simulink library "LIB_TF_G_112"  (Simulink 8.6)
settings: Solver=ode45  StartTime=0.0  StopTime=10.0  RelTol=1e-3
PreLoadFcn:
  | if exist('tl_preloadfcn','file'), tl_preloadfcn(gcs,402); end
PostLoadFcn:
  | if exist('tl_postloadfcn','file'), tl_postloadfcn(gcs,402); end
undefined symbols (not defined in the file or in its folder): ddv
libraries: tllib x2
(part 2 of 2)

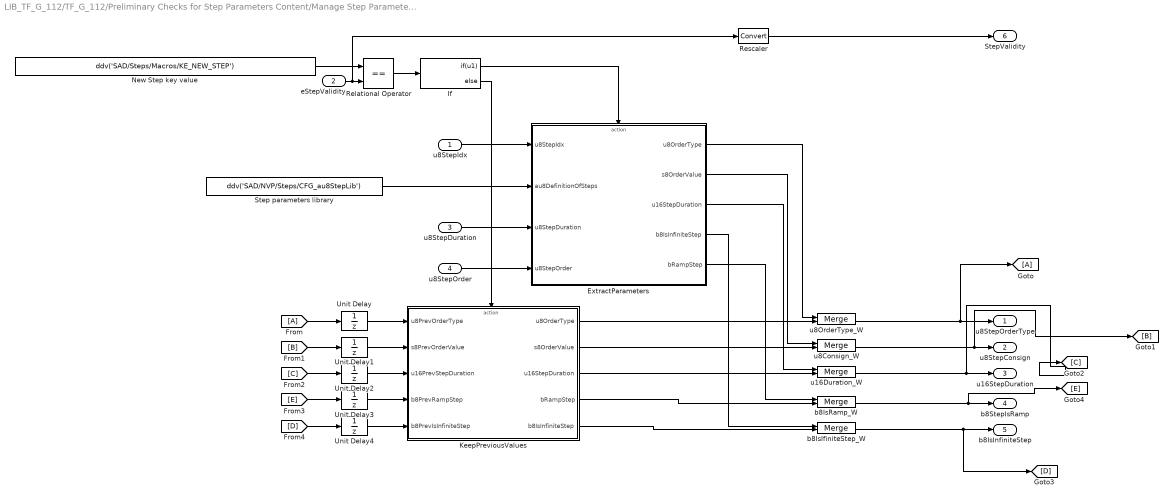
== system LIB_TF_G_112/TF_G_112/Preliminary Checks for Step Parameters Content/Manage Step Parameters ==
  u8StepIdx : Inport
  eStepValidity : Inport  Port=2  PortDimensions=1
  u8StepDuration : Inport  Port=3
  u8StepOrder : Inport  Port=4
  ExtractParameters : Subsystem  RequirementInfo={} %GIDa_f8518a03_50c3_4128_a0d7_e66c9cadc317  TreatAsAtomicUnit=on
  If : If  IfExpression=u1
  KeepPreviousValues : Subsystem  RequirementInfo={} %GIDa_d99f78ca_cceb_45f0_b7aa_f1ab4b729ade  TreatAsAtomicUnit=on
  New Step key value : Constant  Value=ddv('SAD/Steps/Macros/KE_NEW_STEP')  mask(TL_Constant){data={'output',{'variable','SAD/Steps/Macros/KE_NEW_STEP'},'date',738321.40615506948}}
      settings: CopyFcn=if exist('tl_reset_reviewflag','file')==2,tl_reset_reviewflag(gcbh);end  DeleteFcn=if exist('delete_tlblock','file')==2,delete_tlblock(gcbh);end  NameChangeFcn=if exist('rename_tlblock','file')==2,rename_tlblock(gcbh);end  OpenFcn=if exist('tl_open_blockdlg','file')==2,tl_open_blockdlg(gcbh);else,open_system(gcbh,'parameter');end
      mask Help: eval(['if exist(''tl_online_help'',''file'') == 2, tl_online_help(''Topic'',''TL_Constant''),else, web([''jar:file:///'',matlabroot,''/help/toolbox/simulink/help.jar!/slref/' lower(get_param(gcbh,'Blocktype')) '.html''], ''-helpbrowser''),end'])
      mask Display: plot([-0.05, 1.05, NaN, -0.05, 1.05],[.01, .01, NaN, .99, .99])
  Relational Operator : RelationalOperator  Operator===  OutDataTypeStr=boolean  mask(TL_RelationalOperator){data={'date',735951.66826406249}}
      settings: DeleteFcn=if exist('delete_tlblock','file')==2,delete_tlblock(gcbh);end  NameChangeFcn=if exist('rename_tlblock','file')==2,rename_tlblock(gcbh);end  OpenFcn=if exist('tl_open_blockdlg','file')==2,tl_open_blockdlg(gcbh);else,open_system(gcbh,'parameter');end
      mask Help: eval(['if exist(''tl_online_help'',''file'') == 2, tl_online_help(''Topic'',''TL_RelationalOperator''),else, web([''jar:file:///'',matlabroot,''/help/toolbox/simulink/help.jar!/slref/' lower(get_param(gcbh,'Blocktype')) '.html''], ''-helpbrowser''),end'])
      mask Display: plot([-0.05, 1.05, NaN, -0.05, 1.05],[.01, .01, NaN, .99, .99])
  Rescaler : DataTypeConversion  mask(TL_Rescaler){data={'output',{'type','UInt8'},'date',738378.35896812496}}
      settings: DeleteFcn=if exist('delete_tlblock','file')==2,delete_tlblock(gcbh);end  NameChangeFcn=if exist('rename_tlblock','file')==2,rename_tlblock(gcbh);end  OpenFcn=if exist('tl_open_blockdlg','file')==2,tl_open_blockdlg(gcbh);else,open_system(gcbh,'parameter');end
      mask Help: eval(['if exist(''tl_online_help'',''file'') == 2, tl_online_help(''Topic'',''TL_Rescaler''),else, web([''jar:file:///'',matlabroot,''/help/toolbox/simulink/help.jar!/slref/' lower(get_param(gcbh,'Blocktype')) '.html''], ''-helpbrowser''),end'])
      mask Display: plot([-0.1, 1.05, NaN, -0.1, 1.05],[.01, .01, NaN, .99, .99]);
  Step parameters library : Constant  RequirementInfo={} %GIDa_701f29de_2d44_4d45_a297_c60af8fddfb1  Value=ddv('SAD/NVP/Steps/CFG_au8StepLib')  OutDataTypeStr=uint8  SampleTime=-1  mask(TL_Constant){data={'output',{'variable','SAD/NVP/Steps/CFG_au8StepLib'},'date',738321.40645788191}}
      settings: CopyFcn=if exist('tl_reset_reviewflag','file')==2,tl_reset_reviewflag(gcbh);end  DeleteFcn=if exist('delete_tlblock','file')==2,delete_tlblock(gcbh);end  NameChangeFcn=if exist('rename_tlblock','file')==2,rename_tlblock(gcbh);end  OpenFcn=if exist('tl_open_blockdlg','file')==2,tl_open_blockdlg(gcbh);else,open_system(gcbh,'parameter');end
      mask Help: eval(['if exist(''tl_online_help'',''file'') == 2, tl_online_help(''Topic'',''TL_Constant''),else, web([''jar:file:///'',matlabroot,''/help/toolbox/simulink/help.jar!/slref/' lower(get_param(gcbh,'Blocktype')) '.html''], ''-helpbrowser''),end'])
      mask Display: plot([-0.05, 1.05, NaN, -0.05, 1.05],[.01, .01, NaN, .99, .99])
  Unit Delay : UnitDelay  SampleTime=-1  mask(TL_UnitDelay){data={'date',738654.44428931712}}
      settings: CopyFcn=if exist('tl_reset_reviewflag') == 2, tl_reset_reviewflag(gcbh); end  DeleteFcn=if exist('delete_tlblock','file')==2,delete_tlblock(gcbh);end  NameChangeFcn=if exist('rename_tlblock','file')==2,rename_tlblock(gcbh);end  OpenFcn=if exist('tl_open_blockdlg','file')==2,tl_open_blockdlg(gcbh);else,open_system(gcbh,'parameter');end
      mask Help: eval(['if exist(''tl_online_help'',''file'') == 2, tl_online_help(''Topic'',''TL_UnitDelay''),else, web([''jar:file:///'',matlabroot,''/help/toolbox/simulink/help.jar!/slref/' lower(get_param(gcbh,'Blocktype')) '.html''], ''-helpbrowser''),end'])
      mask Display: plot([-0.1, 1.05, NaN, -0.1, 1.05],[.01, .01, NaN, .99, .99]);
  Unit Delay1 : UnitDelay  SampleTime=-1  mask(TL_UnitDelay){data={'date',738654.44460206013}}
      settings: CopyFcn=if exist('tl_reset_reviewflag') == 2, tl_reset_reviewflag(gcbh); end  DeleteFcn=if exist('delete_tlblock','file')==2,delete_tlblock(gcbh);end  NameChangeFcn=if exist('rename_tlblock','file')==2,rename_tlblock(gcbh);end  OpenFcn=if exist('tl_open_blockdlg','file')==2,tl_open_blockdlg(gcbh);else,open_system(gcbh,'parameter');end
      mask Help: eval(['if exist(''tl_online_help'',''file'') == 2, tl_online_help(''Topic'',''TL_UnitDelay''),else, web([''jar:file:///'',matlabroot,''/help/toolbox/simulink/help.jar!/slref/' lower(get_param(gcbh,'Blocktype')) '.html''], ''-helpbrowser''),end'])
      mask Display: plot([-0.1, 1.05, NaN, -0.1, 1.05],[.01, .01, NaN, .99, .99]);
  Unit Delay2 : UnitDelay  SampleTime=-1  mask(TL_UnitDelay){data={'date',738654.44480167818}}
      settings: CopyFcn=if exist('tl_reset_reviewflag') == 2, tl_reset_reviewflag(gcbh); end  DeleteFcn=if exist('delete_tlblock','file')==2,delete_tlblock(gcbh);end  NameChangeFcn=if exist('rename_tlblock','file')==2,rename_tlblock(gcbh);end  OpenFcn=if exist('tl_open_blockdlg','file')==2,tl_open_blockdlg(gcbh);else,open_system(gcbh,'parameter');end
      mask Help: eval(['if exist(''tl_online_help'',''file'') == 2, tl_online_help(''Topic'',''TL_UnitDelay''),else, web([''jar:file:///'',matlabroot,''/help/toolbox/simulink/help.jar!/slref/' lower(get_param(gcbh,'Blocktype')) '.html''], ''-helpbrowser''),end'])
      mask Display: plot([-0.1, 1.05, NaN, -0.1, 1.05],[.01, .01, NaN, .99, .99]);
  Unit Delay3 : UnitDelay  SampleTime=-1  mask(TL_UnitDelay){data={'date',738654.44489355327}}
      settings: CopyFcn=if exist('tl_reset_reviewflag') == 2, tl_reset_reviewflag(gcbh); end  DeleteFcn=if exist('delete_tlblock','file')==2,delete_tlblock(gcbh);end  NameChangeFcn=if exist('rename_tlblock','file')==2,rename_tlblock(gcbh);end  OpenFcn=if exist('tl_open_blockdlg','file')==2,tl_open_blockdlg(gcbh);else,open_system(gcbh,'parameter');end
      mask Help: eval(['if exist(''tl_online_help'',''file'') == 2, tl_online_help(''Topic'',''TL_UnitDelay''),else, web([''jar:file:///'',matlabroot,''/help/toolbox/simulink/help.jar!/slref/' lower(get_param(gcbh,'Blocktype')) '.html''], ''-helpbrowser''),end'])
      mask Display: plot([-0.1, 1.05, NaN, -0.1, 1.05],[.01, .01, NaN, .99, .99]);
  Unit Delay4 : UnitDelay  SampleTime=-1  mask(TL_UnitDelay){data={'date',738654.4449966551}}
      settings: CopyFcn=if exist('tl_reset_reviewflag') == 2, tl_reset_reviewflag(gcbh); end  DeleteFcn=if exist('delete_tlblock','file')==2,delete_tlblock(gcbh);end  NameChangeFcn=if exist('rename_tlblock','file')==2,rename_tlblock(gcbh);end  OpenFcn=if exist('tl_open_blockdlg','file')==2,tl_open_blockdlg(gcbh);else,open_system(gcbh,'parameter');end
      mask Help: eval(['if exist(''tl_online_help'',''file'') == 2, tl_online_help(''Topic'',''TL_UnitDelay''),else, web([''jar:file:///'',matlabroot,''/help/toolbox/simulink/help.jar!/slref/' lower(get_param(gcbh,'Blocktype')) '.html''], ''-helpbrowser''),end'])
      mask Display: plot([-0.1, 1.05, NaN, -0.1, 1.05],[.01, .01, NaN, .99, .99]);
  b8IsIfiniteStep_W : Merge  RequirementInfo={} %GIDa_77d438e3_c130_4039_9d97_7a4272cb0cdf  InitialOutput=ddv('SAD/Vars/Steps/stStep/Components/b8IsPID')  mask(TL_Merge){data={'output',{'variable','SAD/Vars/Steps/stStep/Components/b8IsPID','inheritscaling',0},'date',738342.68413462967}}
      settings: CopyFcn=if exist('tl_reset_reviewflag','file')==2,tl_reset_reviewflag(gcbh);end  DeleteFcn=if exist('delete_tlblock','file')==2,delete_tlblock(gcbh);end  NameChangeFcn=if exist('rename_tlblock','file')==2,rename_tlblock(gcbh);end  OpenFcn=if exist('tl_open_blockdlg','file')==2,tl_open_blockdlg(gcbh);else,open_system(gcbh,'parameter');end
      mask Help: eval(['if exist(''tl_online_help'',''file'') == 2, tl_online_help(''Topic'',''TL_Merge''),else, web([''jar:file:///'',matlabroot,''/help/toolbox/simulink/help.jar!/slref/' lower(get_param(gcbh,'Blocktype')) '.html''], ''-helpbrowser''),end'])
      mask Display: plot([-0.05, 1.05, NaN, -0.05, 1.05],[.01, .01, NaN, .99, .99])
  b8IsRamp_W : Merge  RequirementInfo={} %GIDa_445c0878_ff8b_484e_8dd9_1f96a46135b1  InitialOutput=ddv('SAD/Vars/Steps/stStep/Components/b8IsRamp')  mask(TL_Merge){data={'logdata',{'loggingmode',1},'output',{'variable','SAD/Vars/Steps/stStep/Components/b8IsRamp','inheritscaling',0},'date',738372.37020585651}}
      settings: CopyFcn=if exist('tl_reset_reviewflag','file')==2,tl_reset_reviewflag(gcbh);end  DeleteFcn=if exist('delete_tlblock','file')==2,delete_tlblock(gcbh);end  NameChangeFcn=if exist('rename_tlblock','file')==2,rename_tlblock(gcbh);end  OpenFcn=if exist('tl_open_blockdlg','file')==2,tl_open_blockdlg(gcbh);else,open_system(gcbh,'parameter');end
      mask Help: eval(['if exist(''tl_online_help'',''file'') == 2, tl_online_help(''Topic'',''TL_Merge''),else, web([''jar:file:///'',matlabroot,''/help/toolbox/simulink/help.jar!/slref/' lower(get_param(gcbh,'Blocktype')) '.html''], ''-helpbrowser''),end'])
      mask Display: plot([-0.05, 1.05, NaN, -0.05, 1.05],[.01, .01, NaN, .99, .99])
  u16Duration_W : Merge  RequirementInfo={} %GIDa_ffc47c3a_3ae9_4d19_bffb_b2a8ca4d2a69  InitialOutput=ddv('SAD/Vars/Steps/stStep/Components/u16Duration')  mask(TL_Merge){data={'logdata',{'loggingmode',1},'output',{'variable','SAD/Vars/Steps/stStep/Components/u16Duration','inheritscaling',0},'date',738372.39143710653}}
      settings: CopyFcn=if exist('tl_reset_reviewflag','file')==2,tl_reset_reviewflag(gcbh);end  DeleteFcn=if exist('delete_tlblock','file')==2,delete_tlblock(gcbh);end  NameChangeFcn=if exist('rename_tlblock','file')==2,rename_tlblock(gcbh);end  OpenFcn=if exist('tl_open_blockdlg','file')==2,tl_open_blockdlg(gcbh);else,open_system(gcbh,'parameter');end
      mask Help: eval(['if exist(''tl_online_help'',''file'') == 2, tl_online_help(''Topic'',''TL_Merge''),else, web([''jar:file:///'',matlabroot,''/help/toolbox/simulink/help.jar!/slref/' lower(get_param(gcbh,'Blocktype')) '.html''], ''-helpbrowser''),end'])
      mask Display: plot([-0.05, 1.05, NaN, -0.05, 1.05],[.01, .01, NaN, .99, .99])
  u8Consign_W : Merge  RequirementInfo={} %GIDa_9146a6a1_c3dd_43fd_b49d_8a72e354e92f  InitialOutput=ddv('SAD/Vars/Steps/stStep/Components/u8Consign')  mask(TL_Merge){data={'output',{'variable','SAD/Vars/Steps/stStep/Components/u8Consign','inheritscaling',0},'date',738342.6838825231}}
      settings: CopyFcn=if exist('tl_reset_reviewflag','file')==2,tl_reset_reviewflag(gcbh);end  DeleteFcn=if exist('delete_tlblock','file')==2,delete_tlblock(gcbh);end  NameChangeFcn=if exist('rename_tlblock','file')==2,rename_tlblock(gcbh);end  OpenFcn=if exist('tl_open_blockdlg','file')==2,tl_open_blockdlg(gcbh);else,open_system(gcbh,'parameter');end
      mask Help: eval(['if exist(''tl_online_help'',''file'') == 2, tl_online_help(''Topic'',''TL_Merge''),else, web([''jar:file:///'',matlabroot,''/help/toolbox/simulink/help.jar!/slref/' lower(get_param(gcbh,'Blocktype')) '.html''], ''-helpbrowser''),end'])
      mask Display: plot([-0.05, 1.05, NaN, -0.05, 1.05],[.01, .01, NaN, .99, .99])
  u8OrderType_W : Merge  RequirementInfo={} %GIDa_5609f3d3_6e01_47c8_ab18_eeebdcb5af63  InitialOutput=ddv('SAD/Vars/Steps/stStep/Components/u8Order')  mask(TL_Merge){data={'output',{'variable','SAD/Vars/Steps/stStep/Components/u8Order','inheritscaling',0},'date',738342.6838148958}}
      settings: CopyFcn=if exist('tl_reset_reviewflag','file')==2,tl_reset_reviewflag(gcbh);end  DeleteFcn=if exist('delete_tlblock','file')==2,delete_tlblock(gcbh);end  NameChangeFcn=if exist('rename_tlblock','file')==2,rename_tlblock(gcbh);end  OpenFcn=if exist('tl_open_blockdlg','file')==2,tl_open_blockdlg(gcbh);else,open_system(gcbh,'parameter');end
      mask Help: eval(['if exist(''tl_online_help'',''file'') == 2, tl_online_help(''Topic'',''TL_Merge''),else, web([''jar:file:///'',matlabroot,''/help/toolbox/simulink/help.jar!/slref/' lower(get_param(gcbh,'Blocktype')) '.html''], ''-helpbrowser''),end'])
      mask Display: plot([-0.05, 1.05, NaN, -0.05, 1.05],[.01, .01, NaN, .99, .99])
  u8StepOrderType : Outport
  u8StepConsign : Outport  Port=2
  u16StepDuration : Outport  Port=3
  b8StepIsRamp : Outport  Port=4
  b8IsInfiniteStep : Outport  Port=5
  StepValidity : Outport  Port=6
  wires:
  New Step key value/1 -> Relational Operator/1
  eStepValidity/1 -> Rescaler/1, Relational Operator/2
  Relational Operator/1 -> If/1
  If/2 -> KeepPreviousValues/Action
  u8Consign_W/1 -> [B], u8StepConsign/1
  u16Duration_W/1 -> [C], u16StepDuration/1
  b8IsRamp_W/1 -> [E], b8StepIsRamp/1
  ExtractParameters/1(u8OrderType) -> u8OrderType_W/1
  ExtractParameters/2(s8OrderValue) -> u8Consign_W/1
  ExtractParameters/3(u16StepDuration) -> u16Duration_W/1
  ExtractParameters/5(bRampStep) -> b8IsRamp_W/1
  KeepPreviousValues/1(u8OrderType) -> u8OrderType_W/2
  KeepPreviousValues/2(s8OrderValue) -> u8Consign_W/2
  KeepPreviousValues/3(u16StepDuration) -> u16Duration_W/2
  KeepPreviousValues/4(bRampStep) -> b8IsRamp_W/2
  If/1 -> ExtractParameters/Action
  Step parameters library/1 -> ExtractParameters/2(au8DefinitionOfSteps)
  b8IsIfiniteStep_W/1 -> [D], b8IsInfiniteStep/1
  ExtractParameters/4(b8IsInfiniteStep) -> b8IsIfiniteStep_W/1
  u8StepIdx/1 -> ExtractParameters/1(u8StepIdx)
  u8OrderType_W/1 -> [A], u8StepOrderType/1
  Rescaler/1 -> StepValidity/1
  u8StepDuration/1 -> ExtractParameters/3(u8StepDuration)
  u8StepOrder/1 -> ExtractParameters/4(u8StepOrder)
  [A] -> Unit Delay/1
  [B] -> Unit Delay1/1
  [C] -> Unit Delay2/1
  [D] -> Unit Delay4/1
  [E] -> Unit Delay3/1
  Unit Delay/1 -> KeepPreviousValues/1(u8PrevOrderType)
  Unit Delay1/1 -> KeepPreviousValues/2(s8PrevOrderValue)
  Unit Delay2/1 -> KeepPreviousValues/3(u16PrevStepDuration)
  Unit Delay3/1 -> KeepPreviousValues/4(b8PrevRampStep)
  Unit Delay4/1 -> KeepPreviousValues/5(b8PrevIsInfiniteStep)
  KeepPreviousValues/5(b8IsInfiniteStep) -> b8IsIfiniteStep_W/2

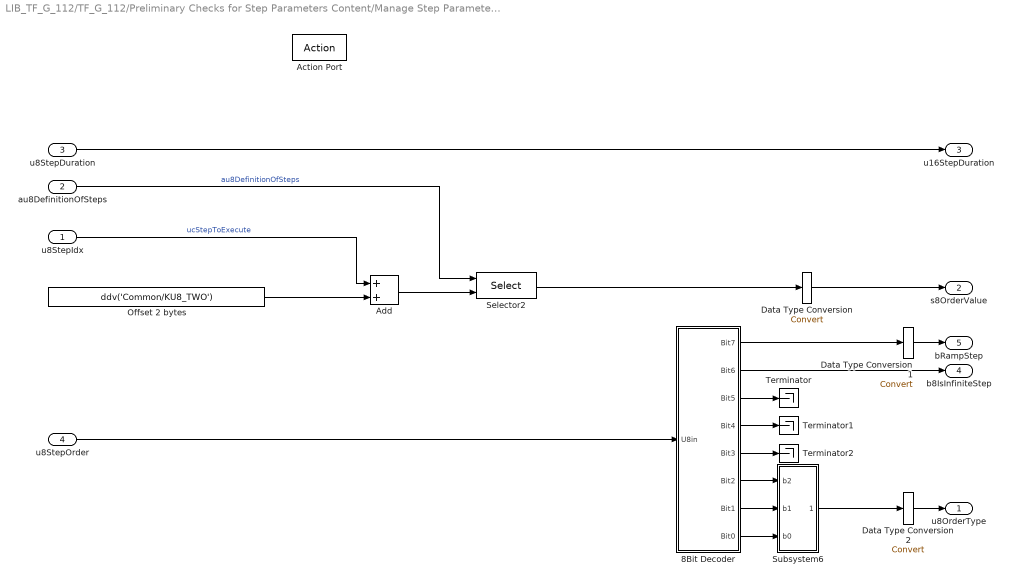
== system LIB_TF_G_112/TF_G_112/Preliminary Checks for Step Parameters Content/Manage Step Parameters/ExtractParameters ==
  u8StepIdx : Inport
  au8DefinitionOfSteps : Inport  RequirementInfo={} %GIDa_5af58792_1cc9_4ce4_bae0_9036b424a801  Port=2
  u8StepDuration : Inport  Port=3
  u8StepOrder : Inport  Port=4
  Action Port : ActionPort  RequirementInfo={} %GIDa_b716945c_1562_44da_9f85_7ecf343fa6e8
  8Bit Decoder : Subsystem  RequirementInfo={} %GIDa_feba0c62_931c_4072_b0ff_45aba4007524  mask(TLSAMPLES_8BIT_DECODER){}
      mask help:
      | Decodes one UInt8 byte into 8 bits.
      | All inputs are boolean variables.
      |
      | Sample implementation using TargetLink Custom Code block.
      | Version 1.0.
  Add : Sum  RequirementInfo={} %GIDa_0a57a462_dd82_4f66_b861_c0720a7e3696  mask(TL_Sum){data={'output',{'name','u16StepByte2','type','UInt16'},'date',735951.66828546301}}
      settings: CopyFcn=if exist('tl_reset_reviewflag','file')==2,tl_reset_reviewflag(gcbh);end  DeleteFcn=if exist('delete_tlblock','file')==2,delete_tlblock(gcbh);end  NameChangeFcn=if exist('rename_tlblock','file')==2,rename_tlblock(gcbh);end  OpenFcn=if exist('tl_open_blockdlg','file')==2,tl_open_blockdlg(gcbh);else,open_system(gcbh,'parameter');end
      mask Help: eval(['if exist(''tl_online_help'',''file'') == 2, tl_online_help(''Topic'',''TL_Sum''),else, web([''jar:file:///'',matlabroot,''/help/toolbox/simulink/help.jar!/slref/' lower(get_param(gcbh,'Blocktype')) '.html''], ''-helpbrowser''),end'])
      mask Display: plot([-0.05, 1.05, NaN, -0.05, 1.05],[.01, .01, NaN, .99, .99])
  Data Type Conversion : DataTypeConversion
  Data Type Conversion1 : DataTypeConversion
  Data Type Conversion2 : DataTypeConversion
  Offset 2 bytes : Constant  RequirementInfo={} %GIDa_19184c90_6870_45c3_8db8_a8942b4be325  Value=ddv('Common/KU8_TWO')  OutDataTypeStr=uint8  SampleTime=-1  mask(TL_Constant){data={'output',{'variable','Common/KU8_TWO'},'date',735951.66827048606}}
      settings: CopyFcn=if exist('tl_reset_reviewflag','file')==2,tl_reset_reviewflag(gcbh);end  DeleteFcn=if exist('delete_tlblock','file')==2,delete_tlblock(gcbh);end  NameChangeFcn=if exist('rename_tlblock','file')==2,rename_tlblock(gcbh);end  OpenFcn=if exist('tl_open_blockdlg','file')==2,tl_open_blockdlg(gcbh);else,open_system(gcbh,'parameter');end
      mask Help: eval(['if exist(''tl_online_help'',''file'') == 2, tl_online_help(''Topic'',''TL_Constant''),else, web([''jar:file:///'',matlabroot,''/help/toolbox/simulink/help.jar!/slref/' lower(get_param(gcbh,'Blocktype')) '.html''], ''-helpbrowser''),end'])
      mask Display: plot([-0.05, 1.05, NaN, -0.05, 1.05],[.01, .01, NaN, .99, .99])
  Selector2 : Selector  RequirementInfo={} %GIDa_4d9cfe24_d7c1_4186_b1de_afe3f89ce847  IndexMode=Zero-based  IndexOptions=Index vector (port)  Indices=[1:10]  OutputSizes=1
  Subsystem6 : Subsystem  RequirementInfo={} %GIDa_5160330e_cdd9_425d_8875_f8236145217b
  Terminator : Terminator
  Terminator1 : Terminator
  Terminator2 : Terminator
  u8OrderType : Outport  RequirementInfo={} %GIDa_a4ff17c9_84cc_43ee_8b0c_3fd6b6f1ed09  InitialOutput=7
  s8OrderValue : Outport  RequirementInfo={} %GIDa_36792c2a_0fa2_493d_8829_1fb3067ac82d  Port=2  InitialOutput=0
  u16StepDuration : Outport  RequirementInfo={} %GIDa_e6c8acc4_bf57_4474_843a_d9aa89ac3819  Port=3  InitialOutput=0
  b8IsInfiniteStep : Outport  RequirementInfo={} %GIDa_2d51edae_6320_46d1_8886_e073955a6cde  Port=4  InitialOutput=0
  bRampStep : Outport  RequirementInfo={} %GIDa_14c0e694_bffc_4663_9ef2_68c7701718bc  Port=5  InitialOutput=0
  wires:
  u8StepIdx/1 -> Add/1  "ucStepToExecute"
  8Bit Decoder/8(Bit0) -> Subsystem6/3(b0)
  8Bit Decoder/7(Bit1) -> Subsystem6/2(b1)
  8Bit Decoder/6(Bit2) -> Subsystem6/1(b2)
  au8DefinitionOfSteps/1 -> Selector2/1  "au8DefinitionOfSteps"
  Offset 2 bytes/1 -> Add/2
  Subsystem6/1(Out1) -> Data Type Conversion2/1
  8Bit Decoder/1(Bit7) -> Data Type Conversion1/1
  Add/1 -> Selector2/2
  Data Type Conversion/1 -> s8OrderValue/1
  Data Type Conversion1/1 -> bRampStep/1
  Data Type Conversion2/1 -> u8OrderType/1
  8Bit Decoder/3(Bit5) -> Terminator/1
  8Bit Decoder/4(Bit4) -> Terminator1/1
  8Bit Decoder/5(Bit3) -> Terminator2/1
  Selector2/1 -> Data Type Conversion/1
  u8StepOrder/1 -> 8Bit Decoder/1(U8in)
  u8StepDuration/1 -> u16StepDuration/1
  8Bit Decoder/2(Bit6) -> b8IsInfiniteStep/1

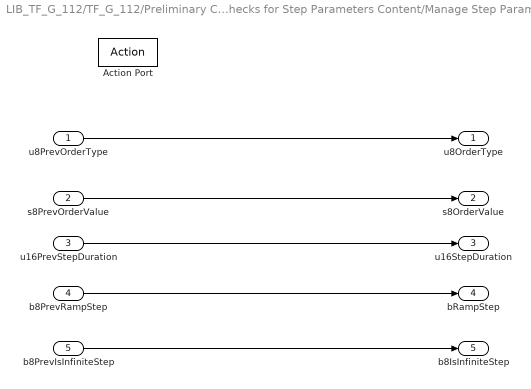
== system LIB_TF_G_112/TF_G_112/Preliminary Checks for Step Parameters Content/Manage Step Parameters/KeepPreviousValues ==
  u8PrevOrderType : Inport  RequirementInfo={} %GIDa_61173a58_4933_4291_992c_59970ace437c
  s8PrevOrderValue : Inport  RequirementInfo={} %GIDa_8cf21477_d934_4301_991e_495f48917b5b  Port=2
  u16PrevStepDuration : Inport  RequirementInfo={} %GIDa_271bfe5f_683d_4e40_816a_3ac303e31e66  Port=3
  b8PrevRampStep : Inport  RequirementInfo={} %GIDa_5931d3fb_f7e2_4f1e_b015_1aa9df9138bb  Port=4
  b8PrevIsInfiniteStep : Inport  RequirementInfo={} %GIDa_2e1a0281_8b1a_4a62_a6b7_d6f3cbbd3bbf  Port=5
  Action Port : ActionPort  RequirementInfo={} %GIDa_96d1ad58_50a9_4027_a59b_05d48c1814fd
  u8OrderType : Outport  RequirementInfo={} %GIDa_fdafd93d_054e_49a8_b09d_e2e4e30d580e  InitialOutput=7
  s8OrderValue : Outport  RequirementInfo={} %GIDa_357db256_5324_4153_8420_788fb44903fc  Port=2  InitialOutput=0
  u16StepDuration : Outport  RequirementInfo={} %GIDa_92a7c2d2_80da_4891_972c_b6d6040a431b  Port=3  InitialOutput=0
  bRampStep : Outport  RequirementInfo={} %GIDa_b542afc9_2a48_4d54_9cbd_42bb43ac3208  Port=4  InitialOutput=0
  b8IsInfiniteStep : Outport  RequirementInfo={} %GIDa_ccc30436_643b_422d_ad64_4a42024accfc  Port=5  InitialOutput=0
  wires:
  b8PrevIsInfiniteStep/1 -> b8IsInfiniteStep/1
  b8PrevRampStep/1 -> bRampStep/1
  u16PrevStepDuration/1 -> u16StepDuration/1
  s8PrevOrderValue/1 -> s8OrderValue/1
  u8PrevOrderType/1 -> u8OrderType/1

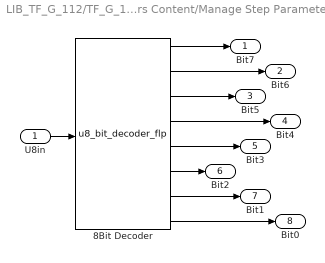
== system LIB_TF_G_112/TF_G_112/Preliminary Checks for Step Parameters Content/Manage Step Parameters/ExtractParameters/8Bit Decoder ==
  U8in : Inport  RequirementInfo={} %GIDa_316296e6_d25f_415d_86a4_ab2f303f2967
  8Bit Decoder : S-Function  RequirementInfo={} %GIDa_81db60bf_2ae0_4350_8dba_f94edd03fe1c  FunctionName=u8_bit_decoder_flp  Parameters=dt  SFunctionDeploymentMode=off  EnableBusSupport=off  mask(TL_CustomCode){data={'#state',0,'#param',0,'#work',0,'#output',8,'#logdata',8,'codefile','u8_bit_decoder.c','output#1',{'name','bIsRampStepRaw','varname','bit7','type','Bool'},'output#2',{'name','$S_$B_bit6','varname','bit6','type','Bool'},'output#3',{'name','bIsReleaseCtrlRaw','varname','bit5','type','Bool'},'output#4',{'name','$S_$B_bit4','varname','bit4','type','Bool'},'output#5',{'name','$S_$B_bit3','varname','bit3','type','Bool'},'output#6',{'name','$S_$B_bit2','varname','bit2','type','Bool'},'output#7',{'name','$S_$B_bit1','varname','bit1','type','Bool'},'output#8',{'name','$S_$B_bit0','varname','bit0','type','Bool'},'input',{'name','$S_$B_in','varname','u8in','type','UInt8'},'date',735951.66829136573}, dt=-1}
      mask help:
      | TargetLink Custom Code block:
      | Allows to insert custom code into a TargetLink application.
      settings: DeleteFcn=if exist('delete_tlblock','file')==2,delete_tlblock(gcbh);end  NameChangeFcn=if exist('rename_tlblock','file')==2,rename_tlblock(gcbh);end  OpenFcn=if exist('tl_open_blockdlg','file')==2,tl_open_blockdlg(gcbh);else,open_system(gcbh,'mask');end
      mask Help: eval('if exist(''tl_online_help'',''file'') == 2, tl_online_help(''Topic'',get_param(gcbh,''MaskType'')),end')
      mask Display:
      | plot([-0.05, 1.05, NaN, -0.05, 1.05],[.01, .01, NaN, .99, .99])
      | ; disp('u8_bit_decoder.c');port_label('input',1,'u8in');port_label('output',1,'bit7');port_label('output',2,'bit6');port_label('output',3,'bit5');port_label('output',4,'bit4');port_label('output',5,'bit3');port_label('output',6,'bit2');port_label('output',7,'bit1');port_label('output',8,'bit0');
  Bit7 : Outport  RequirementInfo={} %GIDa_3e1253f0_2b66_4f5f_9a2b_0a84a073a355
  Bit6 : Outport  RequirementInfo={} %GIDa_a627d821_e196_4b9f_ab67_4eedadb88607  Port=2
  Bit5 : Outport  RequirementInfo={} %GIDa_63315573_79b3_40d9_a8a2_9d817ae078b8  Port=3
  Bit4 : Outport  RequirementInfo={} %GIDa_f646e766_972f_4fff_a2f4_989fa47cfa97  Port=4
  Bit3 : Outport  RequirementInfo={} %GIDa_8223dec1_0264_454d_b26b_ef6deaf87ddf  Port=5
  Bit2 : Outport  RequirementInfo={} %GIDa_adc812c1_ffaa_4134_971e_8e5418b5c1d2  Port=6
  Bit1 : Outport  RequirementInfo={} %GIDa_18117852_57bb_4938_bdc2_0ce63c214a6d  Port=7
  Bit0 : Outport  RequirementInfo={} %GIDa_201e9e1e_c2ed_40b8_a640_dde971076c79  Port=8
  wires:
  U8in/1 -> 8Bit Decoder/1
  8Bit Decoder/6 -> Bit2/1
  8Bit Decoder/1 -> Bit7/1
  8Bit Decoder/2 -> Bit6/1
  8Bit Decoder/3 -> Bit5/1
  8Bit Decoder/4 -> Bit4/1
  8Bit Decoder/5 -> Bit3/1
  8Bit Decoder/7 -> Bit1/1
  8Bit Decoder/8 -> Bit0/1

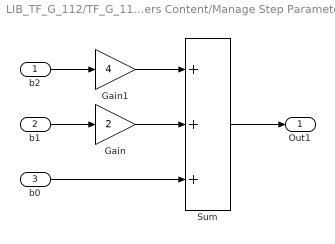
== system LIB_TF_G_112/TF_G_112/Preliminary Checks for Step Parameters Content/Manage Step Parameters/ExtractParameters/Subsystem6 ==
  b2 : Inport  RequirementInfo={} %GIDa_f39ffc53_08bb_4d99_870a_6d3a00ae5965
  b1 : Inport  RequirementInfo={} %GIDa_e32d9dfe_d053_4b46_833a_01c2861930e9  Port=2
  b0 : Inport  RequirementInfo={} %GIDa_b77af5d3_b187_4d2b_b7d3_9ae0d3df018d  Port=3
  Gain : Gain  RequirementInfo={} %GIDa_afc31b96_8064_4e0c_b63a_fe6c51de0fb4  Gain=2  mask(TL_Gain){data={'output',{'type','UInt8'},'date',735951.6682666667}}
      settings: CopyFcn=if exist('tl_reset_reviewflag','file')==2,tl_reset_reviewflag(gcbh);end  DeleteFcn=if exist('delete_tlblock','file')==2,delete_tlblock(gcbh);end  NameChangeFcn=if exist('rename_tlblock','file')==2,rename_tlblock(gcbh);end  OpenFcn=if exist('tl_open_blockdlg','file')==2,tl_open_blockdlg(gcbh);else,open_system(gcbh,'parameter');end
      mask Help: eval(['if exist(''tl_online_help'',''file'') == 2, tl_online_help(''Topic'',''TL_Gain''),else, web([''jar:file:///'',matlabroot,''/help/toolbox/simulink/help.jar!/slref/' lower(get_param(gcbh,'Blocktype')) '.html''], ''-helpbrowser''),end'])
      mask Display: plot([0, .9, 0],[.05, .5, .95])
  Gain1 : Gain  RequirementInfo={} %GIDa_b015b36d_c166_4652_b1a5_ab4222b1e829  Gain=4  mask(TL_Gain){data={'output',{'type','UInt8'},'date',735951.66826613422}}
      settings: CopyFcn=if exist('tl_reset_reviewflag','file')==2,tl_reset_reviewflag(gcbh);end  DeleteFcn=if exist('delete_tlblock','file')==2,delete_tlblock(gcbh);end  NameChangeFcn=if exist('rename_tlblock','file')==2,rename_tlblock(gcbh);end  OpenFcn=if exist('tl_open_blockdlg','file')==2,tl_open_blockdlg(gcbh);else,open_system(gcbh,'parameter');end
      mask Help: eval(['if exist(''tl_online_help'',''file'') == 2, tl_online_help(''Topic'',''TL_Gain''),else, web([''jar:file:///'',matlabroot,''/help/toolbox/simulink/help.jar!/slref/' lower(get_param(gcbh,'Blocktype')) '.html''], ''-helpbrowser''),end'])
      mask Display: plot([0, .9, 0],[.05, .5, .95])
  Sum : Sum  RequirementInfo={'other' '..\..\..\..\Documents and Settings\cedric.sauvage\Desktop\BFE_Design.doc' '@Simulink_requirement_item_4' 'true' 'DSG_BFE_00024' '' } %GIDa_c8ce5980_dba8_42ae_ba5f_36d57ed4039b  Inputs=+++  OutDataTypeStr=uint8  mask(TL_Sum){data={'comment',{'text',['[COVERS: DSG_BFE_00024]'],'placement',2},'output',{'name','u8Order','type','UInt8'},'date',738336.57054458337}}
      settings: CopyFcn=if exist('tl_reset_reviewflag','file')==2,tl_reset_reviewflag(gcbh);end  DeleteFcn=if exist('delete_tlblock','file')==2,delete_tlblock(gcbh);end  NameChangeFcn=if exist('rename_tlblock','file')==2,rename_tlblock(gcbh);end  OpenFcn=if exist('tl_open_blockdlg','file')==2,tl_open_blockdlg(gcbh);else,open_system(gcbh,'parameter');end
      mask Help: eval(['if exist(''tl_online_help'',''file'') == 2, tl_online_help(''Topic'',''TL_Sum''),else, web([''jar:file:///'',matlabroot,''/help/toolbox/simulink/help.jar!/slref/' lower(get_param(gcbh,'Blocktype')) '.html''], ''-helpbrowser''),end'])
      mask Display: plot([-0.05, 1.05, NaN, -0.05, 1.05],[.01, .01, NaN, .99, .99])
  Out1 : Outport  RequirementInfo={} %GIDa_1f355f3a_a679_4013_88c4_dd72188e4f32
  wires:
  Sum/1 -> Out1/1
  b0/1 -> Sum/3
  Gain/1 -> Sum/2
  Gain1/1 -> Sum/1
  b1/1 -> Gain/1
  b2/1 -> Gain1/1
